simulink model "week2_problem3"  (R2020b)
settings: Solver=ode45  StartTime=0.0  StopTime=120.0  RelTol=1e-3
settings Model: DataDictionary=cruise_control.sldd  Creator=gauri  LastModifiedBy=mluser

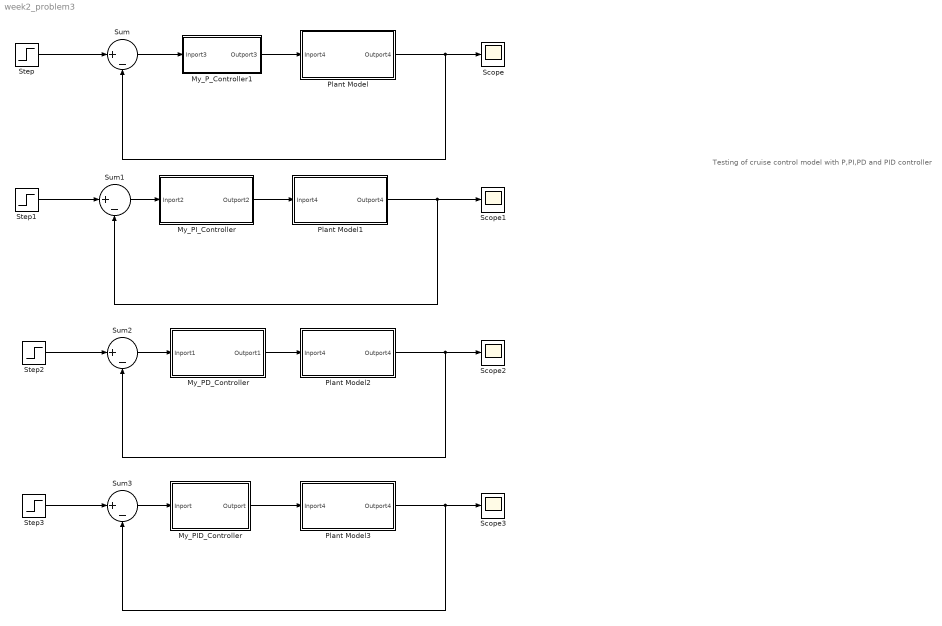
== system week2_problem3 ==
  note: Testing of cruise control model with P,PI,PD and PID controller
  My_PD_Controller : Subsystem  mask{Kp=3545.52783413531, Kd=0}
      mask Display: disp('P.D Controller')
  My_PID_Controller : Subsystem  mask{Kp=424.052164714964, Ki=66.65220823664, Kd=151.936240929117}
      mask Display: disp('P.I.D Controller')
  My_PI_Controller : Subsystem  mask{Kp=338.868980199778, Ki=40.962487388386}
      mask Display: disp('P.I Controller')
  My_P_Controller1 : Subsystem  mask{Kp=491.918085129703}
      mask Display: disp('P Controller')
  Plant Model : Subsystem  mask{m=1000, b=50}
      mask prompts: m "mass"; b "damping"
      mask Display: disp('Cruise Control:Model')
  Plant Model1 : Subsystem  mask{m=1000, b=50}
      mask prompts: m "mass"; b "damping"
      mask Display: disp('Cruise Control:Model')
  Plant Model2 : Subsystem  mask{m=1000, b=50}
      mask prompts: m "mass"; b "damping"
      mask Display: disp('Cruise Control:Model')
  Plant Model3 : Subsystem  mask{m=1000, b=50}
      mask prompts: m "mass"; b "damping"
      mask Display: disp('Cruise Control:Model')
  Scope{,1..3} (4 alike) : Scope
  Step{,1..3} (4 alike) : Step  Time=0  After=500  SampleTime=0
  Sum{,1..3} (4 alike) : Sum  Inputs=|+-
  wires:
  Step/1 -> Sum/1
  Plant Model/1(Outport4) -> Sum/2, Scope/1
  Plant Model1/1(Outport4) -> Sum1/2, Scope1/1
  Step1/1 -> Sum1/1
  Plant Model2/1(Outport4) -> Sum2/2, Scope2/1
  Step2/1 -> Sum2/1
  Step3/1 -> Sum3/1
  Plant Model3/1(Outport4) -> Sum3/2, Scope3/1
  Sum/1 -> My_P_Controller1/1(Inport3)
  My_P_Controller1/1(Outport3) -> Plant Model/1(Inport4)
  Sum1/1 -> My_PI_Controller/1(Inport2)
  My_PI_Controller/1(Outport2) -> Plant Model1/1(Inport4)
  My_PD_Controller/1(Outport1) -> Plant Model2/1(Inport4)
  Sum2/1 -> My_PD_Controller/1(Inport1)
  My_PID_Controller/1(Outport) -> Plant Model3/1(Inport4)
  Sum3/1 -> My_PID_Controller/1(Inport)

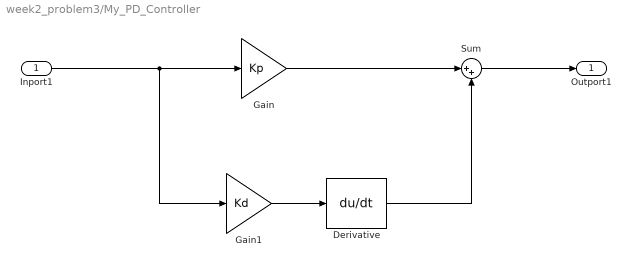
== system week2_problem3/My_PD_Controller ==
  Inport1 : Inport
  Derivative : Derivative
  Gain : Gain  Gain=Kp
  Gain1 : Gain  Gain=Kd
  Sum : Sum  Inputs=|++
  Outport1 : Outport
  wires:
  Derivative/1 -> Sum/2
  Sum/1 -> Outport1/1
  Inport1/1 -> Gain1/1, Gain/1
  Gain1/1 -> Derivative/1
  Gain/1 -> Sum/1

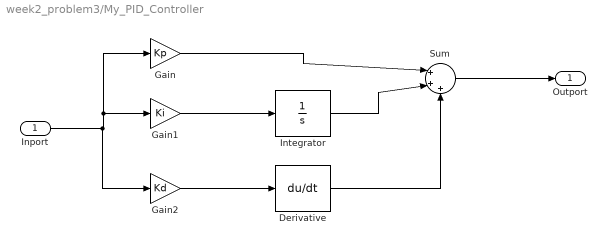
== system week2_problem3/My_PID_Controller ==
  Inport : Inport
  Derivative : Derivative
  Gain : Gain  Gain=Kp
  Gain1 : Gain  Gain=Ki
  Gain2 : Gain  Gain=Kd
  Integrator : Integrator
  Sum : Sum  Inputs=|+++
  Outport : Outport
  wires:
  Sum/1 -> Outport/1
  Gain2/1 -> Derivative/1
  Gain/1 -> Sum/1
  Derivative/1 -> Sum/3
  Gain1/1 -> Integrator/1
  Integrator/1 -> Sum/2
  Inport/1 -> Gain2/1, Gain1/1, Gain/1

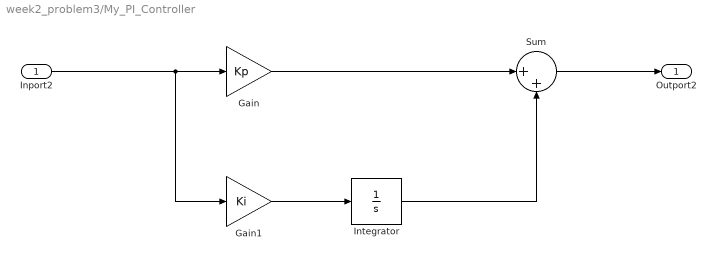
== system week2_problem3/My_PI_Controller ==
  Inport2 : Inport
  Gain : Gain  Gain=Kp
  Gain1 : Gain  Gain=Ki
  Integrator : Integrator
  Sum : Sum  Inputs=|++
  Outport2 : Outport
  wires:
  Integrator/1 -> Sum/2
  Gain/1 -> Sum/1
  Gain1/1 -> Integrator/1
  Sum/1 -> Outport2/1
  Inport2/1 -> Gain1/1, Gain/1

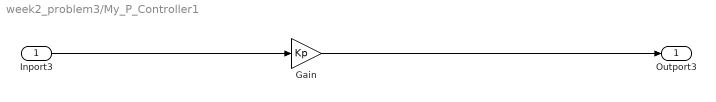
== system week2_problem3/My_P_Controller1 ==
  Inport3 : Inport
  Gain : Gain  Gain=Kp
  Outport3 : Outport
  wires:
  Gain/1 -> Outport3/1
  Inport3/1 -> Gain/1

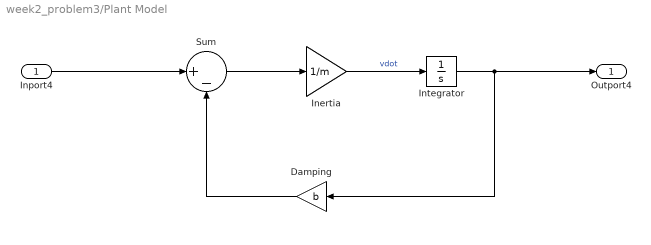
== system week2_problem3/Plant Model ==
  Inport4 : Inport
  Damping : Gain  Gain=b
  Inertia : Gain  Gain=1/m
  Integrator : Integrator
  Sum : Sum  Inputs=|+-
  Outport4 : Outport
  wires:
  Integrator/1 -> Outport4/1, Damping/1
  Damping/1 -> Sum/2
  Inertia/1 -> Integrator/1  "vdot"
  Inport4/1 -> Sum/1
  Sum/1 -> Inertia/1

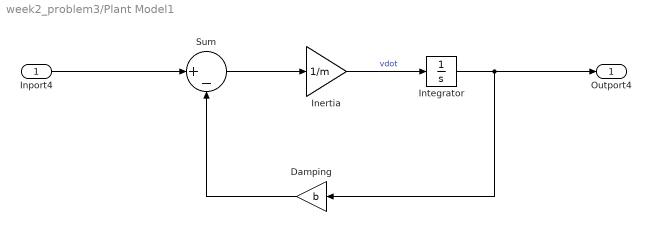
== system week2_problem3/Plant Model1 ==
  Inport4 : Inport
  Damping : Gain  Gain=b
  Inertia : Gain  Gain=1/m
  Integrator : Integrator
  Sum : Sum  Inputs=|+-
  Outport4 : Outport
  wires:
  Integrator/1 -> Outport4/1, Damping/1
  Damping/1 -> Sum/2
  Inertia/1 -> Integrator/1  "vdot"
  Inport4/1 -> Sum/1
  Sum/1 -> Inertia/1

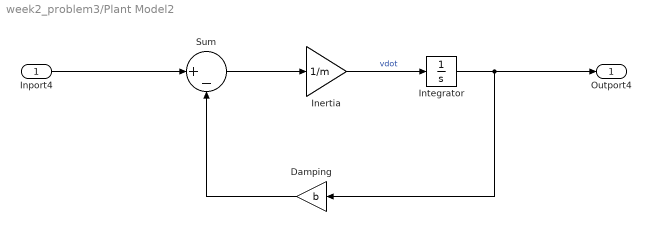
== system week2_problem3/Plant Model2 ==
  Inport4 : Inport
  Damping : Gain  Gain=b
  Inertia : Gain  Gain=1/m
  Integrator : Integrator
  Sum : Sum  Inputs=|+-
  Outport4 : Outport
  wires:
  Integrator/1 -> Outport4/1, Damping/1
  Damping/1 -> Sum/2
  Inertia/1 -> Integrator/1  "vdot"
  Inport4/1 -> Sum/1
  Sum/1 -> Inertia/1

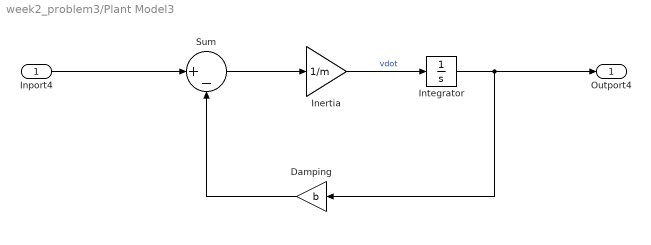
== system week2_problem3/Plant Model3 ==
  Inport4 : Inport
  Damping : Gain  Gain=b
  Inertia : Gain  Gain=1/m
  Integrator : Integrator
  Sum : Sum  Inputs=|+-
  Outport4 : Outport
  wires:
  Integrator/1 -> Outport4/1, Damping/1
  Damping/1 -> Sum/2
  Inertia/1 -> Integrator/1  "vdot"
  Inport4/1 -> Sum/1
  Sum/1 -> Inertia/1
